simulink model "PlantModel"  (R2012b)
settings: Solver=ode45  StartTime=0.0  StopTime=10  RelTol=1e-3
settings Model: Creator=kyle  LastModifiedBy=kyle
settings DataIOCC: InspectSignalLogs=on

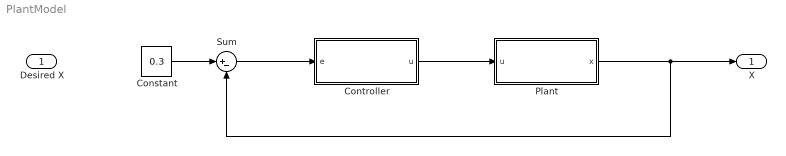
== system PlantModel ==
  Desired X : Inport
  Constant : Constant  Value=0.3
  Controller : Subsystem
  Plant : Subsystem
  Sum : Sum  Inputs=|+-
  X : Outport
  wires:
  Controller/1(u) -> Plant/1(u)
  Constant/1 -> Sum/1
  Sum/1 -> Controller/1(e)
  Plant/1(x) -> Sum/2, X/1

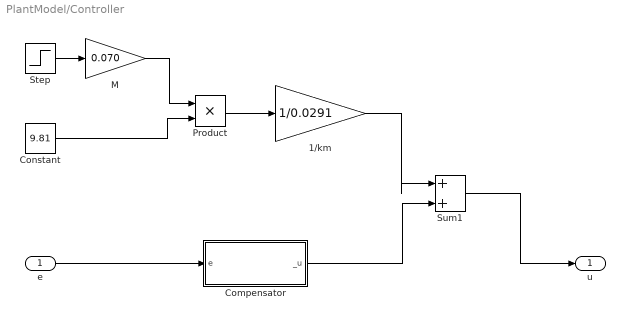
== system PlantModel/Controller ==
  e : Inport
  1/km : Gain  Gain=1/0.0291
  Compensator : Subsystem
  Constant : Constant  Value=9.81
  M : Gain  Gain=0.070
  Product : Product  RndMeth=Zero
  Step : Step  Time=0  SampleTime=0
  Sum1 : Sum  Inputs=|++
  u : Outport
  wires:
  e/1 -> Compensator/1(e)
  Constant/1 -> Product/2
  M/1 -> Product/1
  1/km/1 -> Sum1/1
  Compensator/1(_u) -> Sum1/2
  Sum1/1 -> u/1
  Product/1 -> 1/km/1
  Step/1 -> M/1

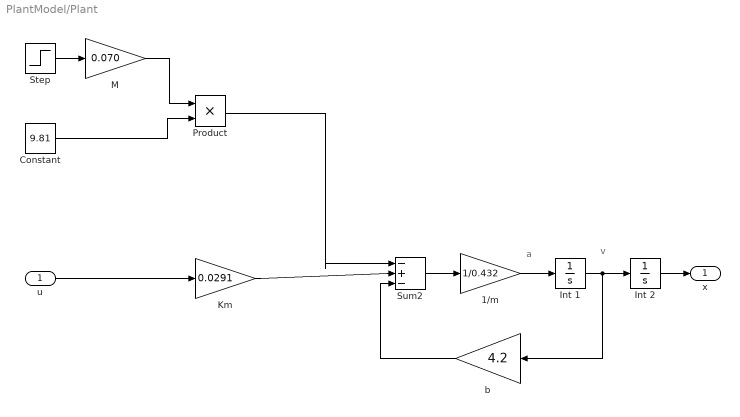
== system PlantModel/Plant ==
  note: a
  note: v
  u : Inport
  1/m : Gain  Gain=1/0.432
  Constant : Constant  Value=9.81
  Int 1 : Integrator
  Int 2 : Integrator
  Km : Gain  Gain=0.0291
  M : Gain  Gain=0.070
  Product : Product  RndMeth=Zero
  Step : Step  Time=0  SampleTime=0
  Sum2 : Sum  Inputs=|-+-
  b : Gain  Gain=4.2
  x : Outport
  wires:
  Km/1 -> Sum2/2
  b/1 -> Sum2/3
  Sum2/1 -> 1/m/1
  Int 1/1 -> b/1, Int 2/1
  Int 2/1 -> x/1
  Product/1 -> Sum2/1
  1/m/1 -> Int 1/1
  u/1 -> Km/1
  Constant/1 -> Product/2
  M/1 -> Product/1
  Step/1 -> M/1

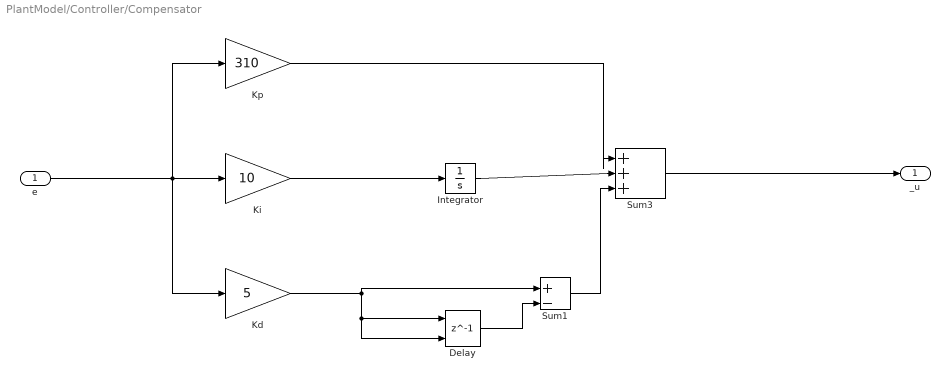
== system PlantModel/Controller/Compensator ==
  e : Inport
  Delay : Delay  DelayLength=1  InitialConditionSource=Input port  InitialCondition=861  InputProcessing=Inherited  SampleTime=.01
      settings: InputPortMap=u0,p4
  Integrator : Integrator
  Kd : Gain  Gain=5
  Ki : Gain  Gain=10
  Kp : Gain  Gain=310
  Sum1 : Sum  Inputs=|+-
  Sum3 : Sum  Inputs=|+++
  _u : Outport
  wires:
  Integrator/1 -> Sum3/2
  Ki/1 -> Integrator/1
  Kp/1 -> Sum3/1
  Sum1/1 -> Sum3/3
  Kd/1 -> Delay/2, Delay/1, Sum1/1
  Delay/1 -> Sum1/2
  Sum3/1 -> _u/1
  e/1 -> Kp/1, Kd/1, Ki/1
